simulink model "controller_dyno"  (R2021b)
settings: Solver=ode15s  StartTime=0.0  StopTime=10000000  MaxStep=2.0  RelTol=1e-3
libraries: slpidlib x2
settings Model: Creator=hitolla  LastModifiedBy=hitolla
settings SolverCC: ZeroCrossAlgorithm=Adaptive
settings DebuggingCC: IgnoredZcDiagnostic=none  UnderSpecifiedDimensionMsg=warning

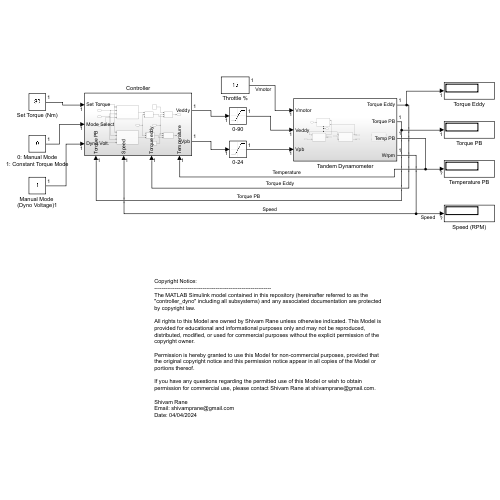
[thumbnail: Simulink's stored preview of the top-level diagram]
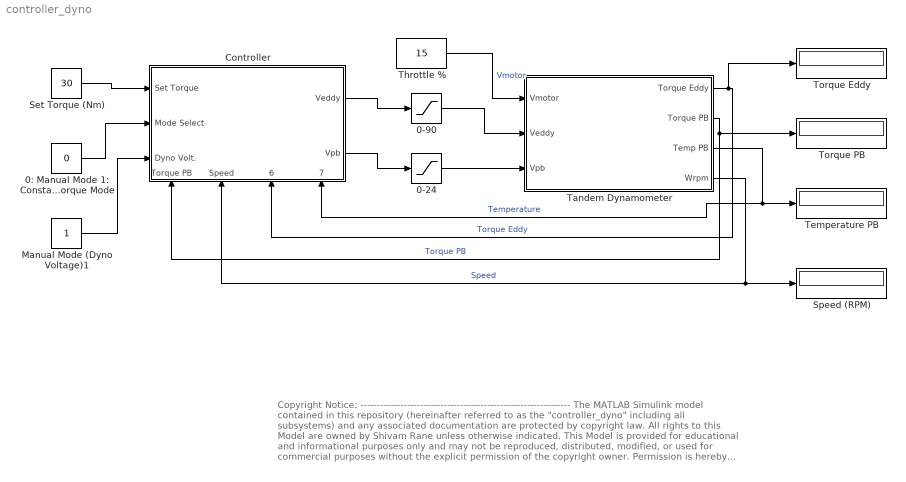
== system controller_dyno ==
  note: Copyright Notice:
      | ---------------------------------------------------------------
      | The MATLAB Simulink model contained in this repository (hereinafter referred to as the "controller_dyno" including all subsystems) and any associated documentation are protected by copyright law.
      |
      | All rights to this Model are owned by Shivam Rane unless otherwise indicated. This Model is provided for educational and informational purposes only and may not be reproduced, distributed, modified, or used for commercial purposes without the explicit permission of the copyright owner.
      |
      | Permission is hereby granted to use this Model for non-commercial purposes, provided that the original copyright notice and this permission notice appear in all copies of the Model or portions thereof.
      |
      | If you have any questions regarding the permitted use of this Model or wish to obtain permission for commercial use, please contact Shivam Rane at shivamprane@gmail.com.
      |
      | Shivam Rane
      | Email: shivamprane@gmail.com
      | Date: 04/04/2024
  0-24 : Saturate  UpperLimit=24  LowerLimit=0
  0-90 : Saturate  UpperLimit=24  LowerLimit=0
  0: Manual Mode 1: Constant Torque Mode : Constant  Value=0
  Controller : Subsystem
      settings: PortSchema="{\"entries\":[{\"content\":{\"sides\":[{\"content\":{\"connectorIds\":[\"In1\",\"In2\",\"In3\"]},\"type\":\"ConnectorPlacement.EquallySpacedRectSide\",\"uuid\":\"e82a3496-e399-455a-af6b-fe4576c39b8e\"},{\"content\":{\"connectorIds\":[\"Out1\",\"Out2\"],\"side\":\"RIGHT\"},\"type\":\"ConnectorPlacement.EquallySpacedRectSide\",\"uuid\":\"65a2a6f4-0c52-49f3-9fc3-064952573b61\"},{\"content\":{\"connectorIds\":[],\"side\":\"TOP\"},\"type\":\"ConnectorPlacement.EquallySpacedRectSide\",\"uuid\":\"c165450a-9074-4547-9939-30c9f7760d0a\"},{\"content\":{\"connectorIds\":[\"In4\",\"In5\",\"In6\",\"In7\"],\"side\":\"BOTTOM\"},\"type\":\"ConnectorPlacement.EquallySpacedRectSide\",\"uuid\":\"2ccff478-9acc-4645-aacb-9b8ba3a6c57d\"}]},\"type\":\"ConnectorPlacement.EquallySpacedConnector\",\"uuid\":\"ec919933-cc4b-44df-bc92-f3a66b3bce33\"}],\"packageUris\":[\"http://schema.mathworks.com/mf0/Connector/R2020b\"],\"version\":\"1.0\"}"
  Manual Mode (Dyno Voltage)1 : Constant
  Set Torque (Nm) : Constant  Value=30
  Speed (RPM) : Display
  Tandem Dynamometer : Subsystem
  Temperature PB : Display
  Throttle % : Constant  Value=15
  Torque Eddy : Display
  Torque PB : Display
  wires:
  Tandem Dynamometer/1(Torque Eddy) -> Controller/6(Torque eddy), Torque Eddy/1  "Torque Eddy"
  Tandem Dynamometer/4(Wrpm) -> Controller/5(Speed), Speed (RPM)/1  "Speed"
  Tandem Dynamometer/2(Torque PB) -> Controller/4(Torque PB), Torque PB/1  "Torque PB"
  Tandem Dynamometer/3(Temp PB) -> Temperature PB/1, Controller/7(Temperature)  "Temperature"
  Set Torque (Nm)/1 -> Controller/1(Set Torque)
  0: Manual Mode 1: Constant Torque Mode/1 -> Controller/2(Mode Select)
  Manual Mode (Dyno Voltage)1/1 -> Controller/3(Dyno Volt.)
  Throttle %/1 -> Tandem Dynamometer/1(Vmotor)  "Vmotor"
  Controller/2(Vpb) -> 0-24/1
  0-24/1 -> Tandem Dynamometer/3(Vpb)
  Controller/1(Veddy) -> 0-90/1
  0-90/1 -> Tandem Dynamometer/2(Veddy)

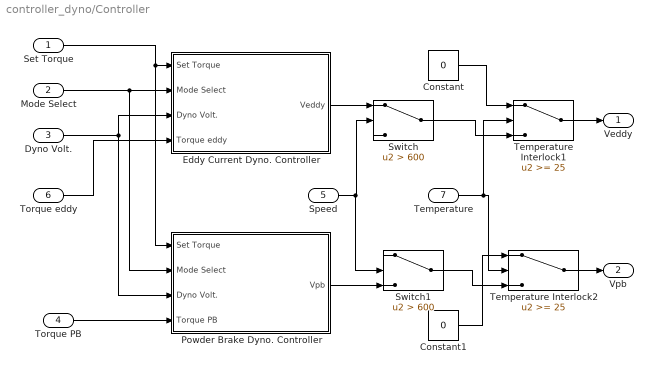
== system controller_dyno/Controller ==
  Set Torque : Inport
  Mode Select : Inport  Port=2
  Dyno Volt. : Inport  Port=3
  Torque PB : Inport  Port=4
  Speed : Inport  Port=5
  Torque eddy : Inport  Port=6
  Temperature : Inport  Port=7
  Constant : Constant  Value=0
  Constant1 : Constant  Value=0
  Eddy Current Dyno. Controller : Subsystem
  Powder Brake Dyno. Controller : Subsystem
  Switch : Switch  Criteria=u2 > Threshold  Threshold=600
  Switch1 : Switch  Criteria=u2 > Threshold  Threshold=600
  Temperature Interlock1 : Switch  Threshold=25
  Temperature Interlock2 : Switch  Threshold=25
  Veddy : Outport
  Vpb : Outport  Port=2
  wires:
  Set Torque/1 -> Powder Brake Dyno. Controller/1(Set Torque), Eddy Current Dyno. Controller/1(Set Torque)
  Mode Select/1 -> Powder Brake Dyno. Controller/2(Mode Select), Eddy Current Dyno. Controller/2(Mode Select)
  Dyno Volt./1 -> Eddy Current Dyno. Controller/3(Dyno Volt.), Powder Brake Dyno. Controller/3(Dyno Volt.)
  Speed/1 -> Switch1/2, Switch/2
  Eddy Current Dyno. Controller/1(Veddy) -> Switch/1
  Powder Brake Dyno. Controller/1(Vpb) -> Switch1/3
  Switch/1 -> Temperature Interlock1/3
  Temperature Interlock1/1 -> Veddy/1
  Switch1/1 -> Temperature Interlock2/3
  Temperature Interlock2/1 -> Vpb/1
  Temperature/1 -> Temperature Interlock1/2, Temperature Interlock2/2
  Constant/1 -> Temperature Interlock1/1
  Constant1/1 -> Temperature Interlock2/1
  Torque eddy/1 -> Eddy Current Dyno. Controller/4(Torque eddy)
  Torque PB/1 -> Powder Brake Dyno. Controller/4(Torque PB)

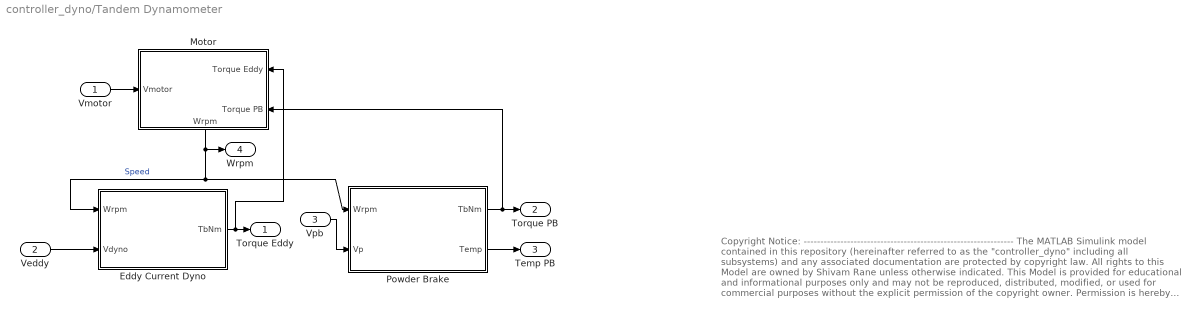
== system controller_dyno/Tandem Dynamometer ==
  note: Copyright Notice:
      | ---------------------------------------------------------------
      | The MATLAB Simulink model contained in this repository (hereinafter referred to as the "controller_dyno" including all subsystems) and any associated documentation are protected by copyright law.
      |
      | All rights to this Model are owned by Shivam Rane unless otherwise indicated. This Model is provided for educational and informational purposes only and may not be reproduced, distributed, modified, or used for commercial purposes without the explicit permission of the copyright owner.
      |
      | Permission is hereby granted to use this Model for non-commercial purposes, provided that the original copyright notice and this permission notice appear in all copies of the Model or portions thereof.
      |
      | If you have any questions regarding the permitted use of this Model or wish to obtain permission for commercial use, please contact Shivam Rane at shivamprane@gmail.com.
      |
      | Shivam Rane
      | Email: shivamprane@gmail.com
      | Date: 04/04/2024
  Vmotor : Inport
  Veddy : Inport  Port=2
  Vpb : Inport  Port=3
  Eddy Current Dyno : Subsystem
  Motor : Subsystem
      settings: PortSchema="{\"entries\":[{\"content\":{\"sides\":[{\"content\":{\"connectorIds\":[\"In1\"]},\"type\":\"ConnectorPlacement.EquallySpacedRectSide\",\"uuid\":\"b326c5d8-ba72-4ed0-b26f-6b1bf398d1d6\"},{\"content\":{\"connectorIds\":[\"In2\",\"In3\"],\"side\":\"RIGHT\"},\"type\":\"ConnectorPlacement.EquallySpacedRectSide\",\"uuid\":\"9cbdfaa4-e8f9-4b5c-8067-0c75074a91af\"},{\"content\":{\"connectorIds\":[],\"side\":\"TOP\"},\"type\":\"ConnectorPlacement.EquallySpacedRectSide\",\"uuid\":\"9f04ae4a-d3e6-4a60-8300-13f25d96c25a\"},{\"content\":{\"connectorIds\":[\"Out1\"],\"side\":\"BOTTOM\"},\"type\":\"ConnectorPlacement.EquallySpacedRectSide\",\"uuid\":\"4f8dda22-8764-4152-b0eb-9176bfd78b8d\"}]},\"type\":\"ConnectorPlacement.EquallySpacedConnector\",\"uuid\":\"8a20e6f4-8832-408b-ab4a-386f53a1b5c3\"}],\"packageUris\":[\"http://schema.mathworks.com/mf0/Connector/R2020b\"],\"version\":\"1.0\"}"
  Powder Brake : Subsystem
  Torque Eddy : Outport
  Torque PB : Outport  Port=2
  Temp PB : Outport  Port=3
  Wrpm : Outport  Port=4
  wires:
  Veddy/1 -> Eddy Current Dyno/2(Vdyno)
  Powder Brake/2(Temp) -> Temp PB/1
  Vpb/1 -> Powder Brake/2(Vp)
  Vmotor/1 -> Motor/1(Vmotor)
  Motor/1(Wrpm) -> Eddy Current Dyno/1(Wrpm), Powder Brake/1(Wrpm), Wrpm/1  "Speed"
  Eddy Current Dyno/1(TbNm) -> Motor/2(Torque Eddy), Torque Eddy/1
  Powder Brake/1(TbNm) -> Motor/3(Torque PB), Torque PB/1

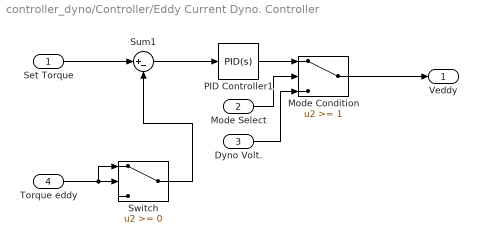
== system controller_dyno/Controller/Eddy Current Dyno. Controller ==
  Set Torque : Inport
  Mode Select : Inport  Port=2
  Dyno Volt. : Inport  Port=3
  Torque eddy : Inport  Port=4
  Mode Condition : Switch  Threshold=1
  PID Controller1 : slpidlib/PID Controller  Controller=PID  Form=Parallel  TimeDomain=Continuous-time  UseExternalTs=off  SampleTime=-1  IntegratorMethod=Forward Euler  FilterMethod=Forward Euler  ControllerParametersSource=internal  P=0.7206  I=13.1386  D=0.0018  UseFilter=on  N=100  TunerSelectOption=Transfer Function Based (PID Tuner App)  InitialConditionSource=internal  InitialConditionForIntegrator=0  InitialConditionForFilter=0  DifferentiatorICPrevScaledInput=0  ExternalReset=none  TrackingMode=off  Kt=1  LimitOutput=off  SatLimitsSource=internal  UpperSaturationLimit=inf  LowerSaturationLimit=-inf  LinearizeAsGain=on  AntiWindupMode=none  Kb=1  POutMin=[]  POutMax=[]  IOutMin=[]  IOutMax=[]  DOutMin=[]  DOutMax=[]  NOutMin=[]  NOutMax=[]  SumOutMin=[]  SumOutMax=[]  SaturationOutMin=[]  SaturationOutMax=[]  PParamMin=[]  PParamMax=[]  IParamMin=[]  IParamMax=[]  DParamMin=[]  DParamMax=[]  NParamMin=[]  NParamMax=[]  KbParamMin=[]  KbParamMax=[]  KtParamMin=[]  KtParamMax=[]  KbOutMin=[]  KbOutMax=[]  KtOutMin=[]  KtOutMax=[]  IntegratorOutMin=[]  IntegratorOutMax=[]  FilterOutMin=[]  FilterOutMax=[]  SumI1OutMin=[]  SumI1OutMax=[]  SumI2OutMin=[]  SumI2OutMax=[]  SumI3OutMin=[]  SumI3OutMax=[]  SumI4OutMin=[]  SumI4OutMax=[]  SumDOutMin=[]  SumDOutMax=[]  DifferentiatorOutMin=[]  DifferentiatorOutMax=[]  FilterDiffOutCoefMin=[]  FilterDiffOutCoefMax=[]  ReciprocalOutMin=[]  ReciprocalOutMax=[]  SumDenOutMin=[]  SumDenOutMax=[]  SumNumOutMin=[]  SumNumOutMax=[]  DivideOutMin=[]  DivideOutMax=[]  UdiffTsProdOutMin=[]  UdiffTsProdOutMax=[]  NTsProdOutMin=[]  NTsProdOutMax=[]  UintegralTsProdOutMin=[]  UintegralTsProdOutMax=[]  UngainTsProdOutMin=[]  UngainTsProdOutMax=[]  IntegratorContinuousStateAttributes=''  IntegratorStateMustResolveToSignalObject=off  IntegratorRTWStateStorageClass=Auto  FilterContinuousStateAttributes=''  FilterStateMustResolveToSignalObject=off  FilterRTWStateStorageClass=Auto  ParallelPVariant=InternalParameters  IdealPVariant=Disabled  IVariant=InternalParameters  DVariant=InternalParameters  IntegratorVariant=Continuous  SatVariant=Disabled  AWVariant=Passthrough  PCopyVariant=Disabled  TRVariant=Disabled  FdbkBlocksVariant=Forward  IdealPFdbkVariant=Disabled  SatFdbkVariant=Disabled  DerivativeFilterVariant=ContFilter  NVariant=InternalParameters  NCopyVariant=Disabled  FilterICVariant=InternalICsFilter  IntegratorICVariant=InternalICs  ExternalResetVariant=Disabled  TRSumVariant=Passthrough  SumFdbkVariant=Disabled  SumVariant=Sum_PID  TsampFilterVariant=InternalTs  TsampNgainVariant=Passthrough  TsampIntegralVariant=Passthrough  ExternalSaturationOutDataTypeStr=Inherit: Same as second input
  Sum1 : Sum  Inputs=|+-
  Switch : Switch
  Veddy : Outport
  wires:
  Sum1/1 -> PID Controller1/1
  Torque eddy/1 -> Switch/1, Switch/2
  Mode Select/1 -> Mode Condition/2
  Mode Condition/1 -> Veddy/1
  Dyno Volt./1 -> Mode Condition/3
  Set Torque/1 -> Sum1/1
  PID Controller1/1 -> Mode Condition/1
  Switch/1 -> Sum1/2

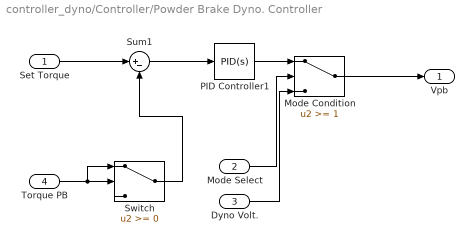
== system controller_dyno/Controller/Powder Brake Dyno. Controller ==
  Set Torque : Inport
  Mode Select : Inport  Port=2
  Dyno Volt. : Inport  Port=3
  Torque PB : Inport  Port=4
  Mode Condition : Switch  Threshold=1
  PID Controller1 : slpidlib/PID Controller  Controller=PID  Form=Parallel  TimeDomain=Continuous-time  UseExternalTs=off  SampleTime=-1  IntegratorMethod=Forward Euler  FilterMethod=Forward Euler  ControllerParametersSource=internal  P=0.7206  I=13.1386  D=0.0018  UseFilter=on  N=100  TunerSelectOption=Frequency Response Based  InitialConditionSource=internal  InitialConditionForIntegrator=0  InitialConditionForFilter=0  DifferentiatorICPrevScaledInput=0  ExternalReset=none  TrackingMode=off  Kt=1  LimitOutput=off  SatLimitsSource=internal  UpperSaturationLimit=inf  LowerSaturationLimit=-inf  LinearizeAsGain=on  AntiWindupMode=none  Kb=1  POutMin=[]  POutMax=[]  IOutMin=[]  IOutMax=[]  DOutMin=[]  DOutMax=[]  NOutMin=[]  NOutMax=[]  SumOutMin=[]  SumOutMax=[]  SaturationOutMin=[]  SaturationOutMax=[]  PParamMin=[]  PParamMax=[]  IParamMin=[]  IParamMax=[]  DParamMin=[]  DParamMax=[]  NParamMin=[]  NParamMax=[]  KbParamMin=[]  KbParamMax=[]  KtParamMin=[]  KtParamMax=[]  KbOutMin=[]  KbOutMax=[]  KtOutMin=[]  KtOutMax=[]  IntegratorOutMin=[]  IntegratorOutMax=[]  FilterOutMin=[]  FilterOutMax=[]  SumI1OutMin=[]  SumI1OutMax=[]  SumI2OutMin=[]  SumI2OutMax=[]  SumI3OutMin=[]  SumI3OutMax=[]  SumI4OutMin=[]  SumI4OutMax=[]  SumDOutMin=[]  SumDOutMax=[]  DifferentiatorOutMin=[]  DifferentiatorOutMax=[]  FilterDiffOutCoefMin=[]  FilterDiffOutCoefMax=[]  ReciprocalOutMin=[]  ReciprocalOutMax=[]  SumDenOutMin=[]  SumDenOutMax=[]  SumNumOutMin=[]  SumNumOutMax=[]  DivideOutMin=[]  DivideOutMax=[]  UdiffTsProdOutMin=[]  UdiffTsProdOutMax=[]  NTsProdOutMin=[]  NTsProdOutMax=[]  UintegralTsProdOutMin=[]  UintegralTsProdOutMax=[]  UngainTsProdOutMin=[]  UngainTsProdOutMax=[]  IntegratorContinuousStateAttributes=''  IntegratorStateMustResolveToSignalObject=off  IntegratorRTWStateStorageClass=Auto  FilterContinuousStateAttributes=''  FilterStateMustResolveToSignalObject=off  FilterRTWStateStorageClass=Auto  ParallelPVariant=InternalParameters  IdealPVariant=Disabled  IVariant=InternalParameters  DVariant=InternalParameters  IntegratorVariant=Continuous  SatVariant=Disabled  AWVariant=Passthrough  PCopyVariant=Disabled  TRVariant=Disabled  FdbkBlocksVariant=Forward  IdealPFdbkVariant=Disabled  SatFdbkVariant=Disabled  DerivativeFilterVariant=ContFilter  NVariant=InternalParameters  NCopyVariant=Disabled  FilterICVariant=InternalICsFilter  IntegratorICVariant=InternalICs  ExternalResetVariant=Disabled  TRSumVariant=Passthrough  SumFdbkVariant=Disabled  SumVariant=Sum_PID  TsampFilterVariant=InternalTs  TsampNgainVariant=Passthrough  TsampIntegralVariant=Passthrough  ExternalSaturationOutDataTypeStr=Inherit: Same as second input
  Sum1 : Sum  Inputs=|+-
  Switch : Switch
  Vpb : Outport
  wires:
  Torque PB/1 -> Switch/1, Switch/2
  Mode Select/1 -> Mode Condition/2
  Mode Condition/1 -> Vpb/1
  Dyno Volt./1 -> Mode Condition/3
  Set Torque/1 -> Sum1/1
  Switch/1 -> Sum1/2
  PID Controller1/1 -> Mode Condition/1
  Sum1/1 -> PID Controller1/1

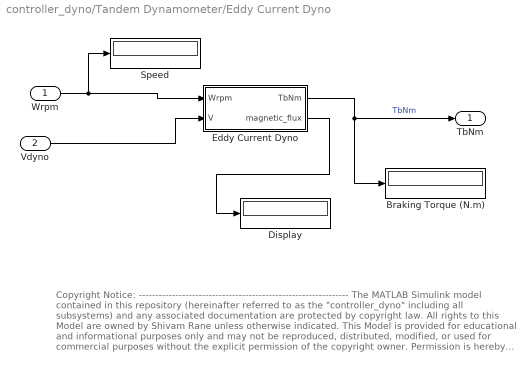
== system controller_dyno/Tandem Dynamometer/Eddy Current Dyno ==
  note: Copyright Notice:
      | ---------------------------------------------------------------
      | The MATLAB Simulink model contained in this repository (hereinafter referred to as the "controller_dyno" including all subsystems) and any associated documentation are protected by copyright law.
      |
      | All rights to this Model are owned by Shivam Rane unless otherwise indicated. This Model is provided for educational and informational purposes only and may not be reproduced, distributed, modified, or used for commercial purposes without the explicit permission of the copyright owner.
      |
      | Permission is hereby granted to use this Model for non-commercial purposes, provided that the original copyright notice and this permission notice appear in all copies of the Model or portions thereof.
      |
      | If you have any questions regarding the permitted use of this Model or wish to obtain permission for commercial use, please contact Shivam Rane at shivamprane@gmail.com.
      |
      | Shivam Rane
      | Email: shivamprane@gmail.com
      | Date: 04/04/2024
  Wrpm : Inport
  Vdyno : Inport  Port=2
  Braking Torque (N.m) : Display
  Display : Display
  Eddy Current Dyno : MATLAB Function  TreatAsAtomicUnit=on
  Speed : Display
  TbNm : Outport
  wires:
  Eddy Current Dyno/1(TbNm) -> TbNm/1, Braking Torque (N.m)/1  "TbNm"
  Wrpm/1 -> Speed/1, Eddy Current Dyno/1(Wrpm)
  Vdyno/1 -> Eddy Current Dyno/2(V)
  Eddy Current Dyno/2(magnetic_flux) -> Display/1

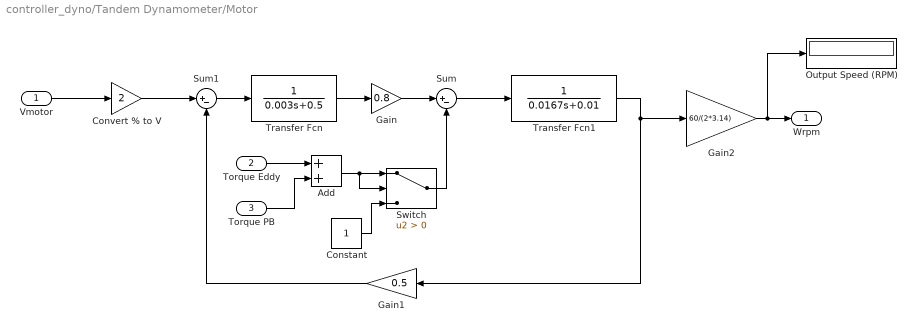
== system controller_dyno/Tandem Dynamometer/Motor ==
  Vmotor : Inport
  Torque Eddy : Inport  Port=2
  Torque PB : Inport  Port=3
  Add : Sum
  Constant : Constant
  Convert % to V : Gain  Gain=2
  Gain : Gain  Gain=0.8
  Gain1 : Gain  Gain=0.5
  Gain2 : Gain  Gain=60/(2*3.14)
  Output Speed (RPM) : Display
  Sum : Sum  Inputs=|+-
  Sum1 : Sum  Inputs=|+-
  Switch : Switch  Criteria=u2 > Threshold
  Transfer Fcn : TransferFcn  Denominator=[0.003 0.5]
  Transfer Fcn1 : TransferFcn  Denominator=[0.0167 0.01]  ParameterTunability=Optimized
  Wrpm : Outport
  wires:
  Transfer Fcn/1 -> Gain/1
  Gain/1 -> Sum/1
  Sum/1 -> Transfer Fcn1/1
  Sum1/1 -> Transfer Fcn/1
  Gain1/1 -> Sum1/2
  Constant/1 -> Switch/3
  Switch/1 -> Sum/2
  Gain2/1 -> Output Speed (RPM)/1, Wrpm/1
  Transfer Fcn1/1 -> Gain1/1, Gain2/1
  Convert % to V/1 -> Sum1/1
  Vmotor/1 -> Convert % to V/1
  Add/1 -> Switch/2, Switch/1
  Torque Eddy/1 -> Add/1
  Torque PB/1 -> Add/2

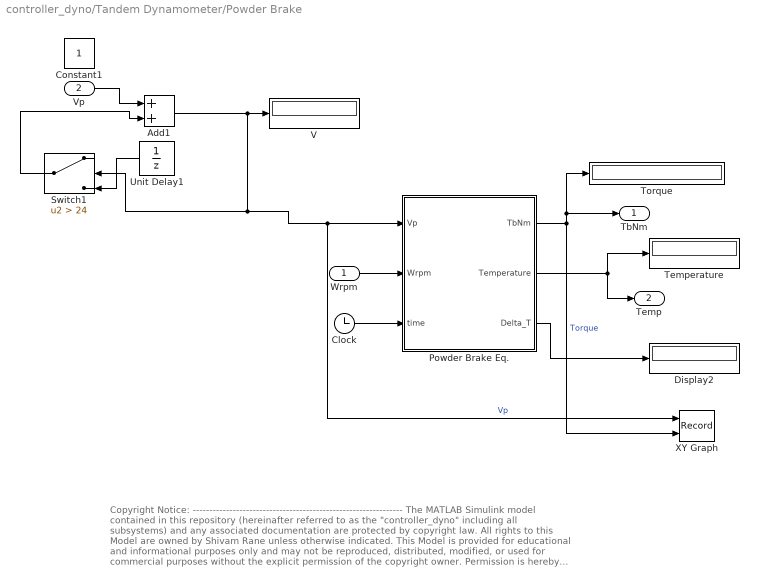
== system controller_dyno/Tandem Dynamometer/Powder Brake ==
  note: Copyright Notice:
      | ---------------------------------------------------------------
      | The MATLAB Simulink model contained in this repository (hereinafter referred to as the "controller_dyno" including all subsystems) and any associated documentation are protected by copyright law.
      |
      | All rights to this Model are owned by Shivam Rane unless otherwise indicated. This Model is provided for educational and informational purposes only and may not be reproduced, distributed, modified, or used for commercial purposes without the explicit permission of the copyright owner.
      |
      | Permission is hereby granted to use this Model for non-commercial purposes, provided that the original copyright notice and this permission notice appear in all copies of the Model or portions thereof.
      |
      | If you have any questions regarding the permitted use of this Model or wish to obtain permission for commercial use, please contact Shivam Rane at shivamprane@gmail.com.
      |
      | Shivam Rane
      | Email: shivamprane@gmail.com
      | Date: 04/04/2024
  Wrpm : Inport
  Vp : Inport  Port=2
  Add1 : Sum
  Clock : Clock
  Constant1 : Constant
  Display2 : Display
  Powder Brake Eq. : MATLAB Function  TreatAsAtomicUnit=on
  Switch1 : Switch  Criteria=u2 > Threshold  Threshold=24
  Temperature : Display
  Torque : Display
  Unit Delay1 : UnitDelay  SampleTime=10000  HasFrameUpgradeWarning=on
  V : Display
  XY Graph : Record  FileSettingsInternal="{\"entries\":[{\"content\":{\"excelSettings\":{\"content\":{},\"type\":\"Streamout.ExcelSettings\"}},\"type\":\"Streamout.FileSettingStorage\",\"uuid\":\"9a5bce44-44d7-4340-837c-82606f0fa55a\"}],\"packageUris\":[\"http://schema.mathworks.com/mf0/streamout_blocks/R2020a\"],\"version\":\"1.0\"}"  Layout=[1 1]  SignalsInternal="{\"entries\":[{\"content\":{\"signals\":[{\"content\":{\"blockPath\":[\"controller_dyno/Tandem Dynamometer/Powder Brake/XY Graph\"],\"channel\":[],\"dimensions\":[1],\"domain\":\"controller_dyno/Tandem Dynamometer/Powder Brake/XY Graph\",\"lineColor\":\"#ff6929\",\"plots\":[],\"port\":1,\"sid\":[],\"signalID\":9,\"signalName\":\"Vp\"},\"type\":\"RecordBlkView.Signal\",\"uuid\":\"9ab077b7-73b6-430b-b8f2-c30c711ec71d\"},{\"content\":{\"blockPath\":[\"controller_dyno/Tandem Dynamometer/Powder Brake/XY Graph\"],\"channel\":[],\"dimensions\":[1],\"domain\":\"controller_dyno/Tandem Dynamometer/Powder Brake/XY Graph\",\"lineColor\":\"#b746ff\",\"plots\":[],\"port\":2,\"sid\":[],\"signalID\":12,\"signalName\":\"Torque\"},\"type\":\"RecordBlkView.Signal\",\"uuid\":\"9ddcbb86-e421-47aa-875c-d6e60fd9389d\"}]},\"type\":\"RecordBlkView.InputSignals\",\"uuid\":\"5ea54850-cd8b-452e-abb5-19360d75a008\"}],\"packageUris\":[\"http://schema.mathworks.com/mf0/streamout_blocks/R2020a\"],\"version\":\"1.0\"}"  VisualizationBindings="{\"xyplotplugin\":{\"info\":[{\"series\":[],\"subplotID\":1}]}}"  CompatibilityTag=XY
  TbNm : Outport
  Temp : Outport  Port=2
  wires:
  Powder Brake Eq./1(TbNm) -> XY Graph/2, TbNm/1, Torque/1  "Torque"
  Clock/1 -> Powder Brake Eq./3(time)
  Powder Brake Eq./3(Delta_T) -> Display2/1
  Add1/1 -> V/1, Switch1/2, XY Graph/1, Powder Brake Eq./1(Vp)  "Vp"
  Unit Delay1/1 -> Switch1/3
  Switch1/1 -> Add1/2
  Powder Brake Eq./2(Temperature) -> Temperature/1, Temp/1
  Wrpm/1 -> Powder Brake Eq./2(Wrpm)
  Vp/1 -> Add1/1

== matlab function controller_dyno/Tandem Dynamometer/Eddy Current Dyno/Eddy Current Dyno ==
  data: Wrpm input; TbNm output; V input; magnetic_flux output
function [TbNm,magnetic_flux]= fcn(Wrpm, V)

% "Numerical_Data" refers to the design parameters of the Dynamometer

r = "Numerical_Data";% Radius(mm): Round core condidered 
A = 3.14*r*r; % Area (mm2)

% Rotating disk parameters
d = "Numerical_Data"; % Thickness of rotating disk (mm)
a = "Numerical_Data"; % distance from rotating center to the center of pole shoe (mm)
Po = "Numerical_Data"; % Electric Resistivity of rotating disk
alpha = 300/1000;
Temp = "Numerical_Data"; % Temperature (degree celcius)
Elec_Cond = 1/(Po*(1+alpha*Temp)); % Electric Conductivity of rotating disk


Ur = "Numerical_Data"; % Relative Permeability
Uo = (4*3.14)/10000000; % Relative permiability of core
lg = "Numerical_Data"; % Distance between pole shoes (mm)

Ra = (lg - d)/(Uo*A); % Magnetic reluctance of air-gap
Rd = d/(Ur*Uo*A); % Magnetic reluctance of rotating disk
Rg = Ra+Rd; % Reluctance outside the core


W = Wrpm*((2*3.14)/60); % speed in rad
N = "Numerical_Data"; % number of turns of the coil
I = (8*V)/90; % currrent in the range of 0 to 8 A

magnetic_flux = (N*I)/(Ra + (Elec_Cond*a*d*r*(W/A)));

Bc = magnetic_flux/A; % Coil-core magnetic flux density
Bsat = 1.5;
Ncoil = "Numerical_Data";

Je = Elec_Cond*a*(W*Bc); % Current density of eddy current induced at pole
Pd = Ncoil*Je*Je*A*d; % power dissipated
TbNmm = Pd/W; % Braking Torque (N.mm)
Error = "Numerical_Data"; %Error torque (if any)
TbNm = (TbNmm/1000)+Error; % Braking Torque (N.m)

== matlab function controller_dyno/Tandem Dynamometer/Powder Brake/Powder Brake Eq. ==
  data: TbNm output; Vp input; Wrpm input; Temperature output; time input; Delta_T output
function [TbNm, Temperature, Delta_T]= fcn(Vp,Wrpm,time)

% "Numerical_Data" refers to the design parameters of the Dynamometer

N = "Numerical_Data"; % number of turns of the coil
I = (5*Vp)/24; % currrent in the range of 0 to 8 A


w = "Numerical_Data"; % disc width (mm)
Dd = "Numerical_Data"; % disc outer diameter (mm)
Dc = "Numerical_Data"; % inner diameter of coil body

rd = Dd/2; % disc outer radius (mm)
rc = Dc/2; % inner radius of coil body
Gc = rc-rd; % Gap width

Ad = 3.14*rd*rd; % cross sectional Area of disc

Disc_circumference = 2*3.14*rd; 

Ads = 2*3.14*rd*w; % Lateral Surface area of disc circumference (sq.mm)
Uo = 0.00000126; % Permiability of Vacuum (T/m)

Magnetic_Field_Point = (Uo*N*I)/(2*3.14*Gc); % Magnetic Field (T)

Magnetic_Field_Total = Magnetic_Field_Point*Disc_circumference;

Fc = "Numerical_Data"; % Friction coeff. of iron powder and MS
Friction_force = Magnetic_Field_Total*Fc; % Friction force (N)

Tf = Friction_force*Disc_circumference*w;
Er = "Numerical_Data"; %Error Torque (if any)
TbNm = ((Tf*rd)/1000)+Er; % Torque (Nm)

W = ((2*3.14*Wrpm)/60); % speed in rad


%         Temperaure
time_Min = time/60;

Q = (2*3.14*TbNm*W*time_Min); % heat generated from torque

Density_MS = 0.00000785; % Density of mild steel in g/mm^3

m = (Density_MS*Ad*w); % mass
c = 420; % specific heat capacity
Ambient_Temp = 24; % degree C
Delta_T = Q/(m*c*Ads); % Temperature change in degree C

Temperature = Ambient_Temp + Delta_T; % Temperature in degree C
